simulink model "requirements"  (R2022a)
settings: Solver=FixedStepAuto  StartTime=0.0  StopTime=10.0  FixedStep=1e-3  RelTol=1e-3  EnableMultiTasking=on
settings Model: ExtModeTrigDuration=5  Creator=zaree  LastModifiedBy=zaree
settings OptimizationCC: EnhancedBackFolding=on  PassReuseOutputArgsAs=Individual arguments  ZeroExternalMemoryAtStartup=off  ZeroInternalMemoryAtStartup=off  MaxStackSize=64  OptimizeBlockOrder=speed  DifferentSizesBufferReuse=on  OptimizationCustomize=off  EfficientTunableParamExpr=on
settings DebuggingCC: ParameterTunabilityLossMsg=error
settings HardwareCC: ProdBitPerPointer=32  ProdBitPerSizeT=32  ProdBitPerPtrDiffT=32  ProdLargestAtomicInteger=Long  ProdLargestAtomicFloat=Double  ProdWordSize=32  ProdHWDeviceType=ARM Compatible->ARM Cortex
settings SFSimCC: MATLABDynamicMemAlloc=off
settings RTWCC: SystemTargetFile=ert.tlc  HardwareBoard=NXP FRDM-K64F  TLCOptions="-aInlineSetEventsForThisBaseRateFcn=TLC_FALSE -aSuppressMultiTaskScheduler=TLC_FALSE  -aRateBasedStepFcn=0"  TemplateMakefile=ert_default_tmf  Toolchain=GNU Tools for ARM Embedded Processors
settings CodeAppCC: ForceParamTrailComments=on  IgnoreCustomStorageClasses=off  OperatorAnnotations=on  SimulinkDataObjDesc=on  SFDataObjDesc=on  InsertBlockDesc=on
settings ERTTargetCC: ExtModeTransport=4  ExtModeMexFile=sendToCommService

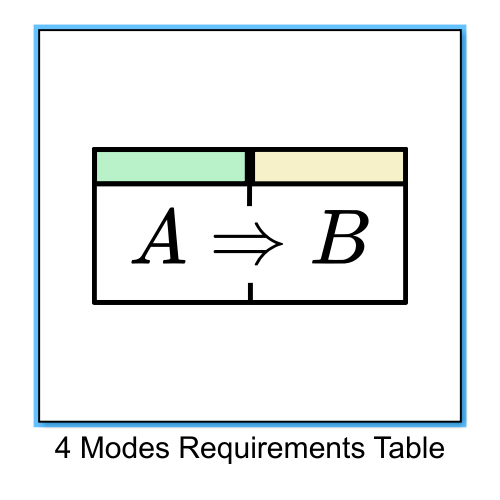
[thumbnail: Simulink's stored preview of the top-level diagram]
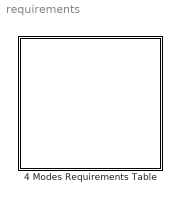
== system requirements ==
  4 Modes Requirements Table : Requirements Table  TreatAsAtomicUnit=on

== stateflow chart requirements/4 Modes Requirements Table ==
  (default) -> (junction 1073742873)
  (junction 1073742873) -> (junction 1073742874) : {
      | % SF_REQ_REV_07
      | }
  (junction 1073742874) -> (junction 1073742876) : {
      | % HEADER_ASSIGNMENTS
      |
      | }
  (junction 1073742876) -> (junction 1073742878) : {
      | % START_A_4
      | }
  (junction 1073742878) -> (junction 1073742880) : {
      | }
  (junction 1073742880) -> (junction 1073742882)
  (junction 1073742882) -> (junction 1073742884) : {
      | }
  (junction 1073742884) -> (junction 1073742886) : {
      | % END_A_4
      | }
  (junction 1073742886) -> (junction 1073742888) : {
      | % START_R_1
      | }
  (junction 1073742888) -> (junction 1073742890) : {
      | }
  (junction 1073742890) -> (junction 1073742892)
  (junction 1073742892) -> (junction 1073742894) [order 1] : [duration((PACE_CHARGE_CTRL == 0) && (ATR_CHARGE_CTRL == 1) && (ATR_GND_CTRL == 0) && (PACE_GND_CTRL == 1) && (Z_ATR_CTRL == 0)) >= LRI-Atrial_Pulse_Width]
  (junction 1073742892) -> (junction 1073742900) [order 2]
  (junction 1073742894) -> (junction 1073742896) : {
      | reqtable_postcondition((PACE_CHARGE_CTRL == 1) && (ATR_PACE_CTRL == 0) && (ATR_GND_CTRL == 1) && (PACE_GND_CTRL == 1) && (Z_ATR_CTRL == 0), 'R:1');
      |
      |
      | }
  (junction 1073742896) -> (junction 1073742898) : {
      | }
  (junction 1073742898) -> (junction 1073742900)
  (junction 1073742900) -> (junction 1073742902)
  (junction 1073742902) -> (junction 1073742904) : {
      | % END_R_1
      | }
  (junction 1073742904) -> (junction 1073742906) : {
      | % START_R_7
      | }
  (junction 1073742906) -> (junction 1073742908) : {
      | }
  (junction 1073742908) -> (junction 1073742910)
  (junction 1073742910) -> (junction 1073742912) [order 1] : [duration((PACE_CHARGE_CTRL == 1) && (ATR_PACE_CTRL==0) && (ATR_GND_CTRL==1) && (PACE_GND_CTRL == 1) && (Z_ATR_CTRL == 0)) >= Atrial_Pulse_Width]
  (junction 1073742910) -> (junction 1073742918) [order 2]
  (junction 1073742912) -> (junction 1073742914) : {
      | reqtable_postcondition((PACE_CHARGE_CTRL == 0) && (ATR_CHARGE_CTRL == 1) && (ATR_GND_CTRL == 0) && (PACE_GND_CTRL == 1) && (Z_ATR_CTRL == 0), 'R:2');
      |
      |
      | }
  (junction 1073742914) -> (junction 1073742916) : {
      | }
  (junction 1073742916) -> (junction 1073742918)
  (junction 1073742918) -> (junction 1073742920)
  (junction 1073742920) -> (junction 1073742922) : {
      | % END_R_7
      | }
  (junction 1073742922) -> (junction 1073742924) : {
      | % START_R_10
      | }
  (junction 1073742924) -> (junction 1073742926) : {
      | }
  (junction 1073742926) -> (junction 1073742928)
  (junction 1073742928) -> (junction 1073742930) [order 1] : [duration((PACE_CHARGE_CTRL == 0) && (VENT_PACE_CTRL == 1) && (VENT_GND_CTRL == 0) && (PACE_GND_CTRL == 1) && (Z_VENT_CTRL == 0)) >= LRI-Ventricular_Pulse_Width]
  (junction 1073742928) -> (junction 1073742936) [order 2]
  (junction 1073742930) -> (junction 1073742932) : {
      | reqtable_postcondition((PACE_CHARGE_CTRL == 1) && (VENT_CHARGE_CTRL == 0) && (VENT_GND_CTRL == 1) && (PACE_GND_CTRL == 1) && (Z_VENT_CTRL == 0), 'R:3');
      |
      |
      | }
  (junction 1073742932) -> (junction 1073742934) : {
      | }
  (junction 1073742934) -> (junction 1073742936)
  (junction 1073742936) -> (junction 1073742938)
  (junction 1073742938) -> (junction 1073742940) : {
      | % END_R_10
      | }
  (junction 1073742940) -> (junction 1073742942) : {
      | % START_R_13
      | }
  (junction 1073742942) -> (junction 1073742944) : {
      | }
  (junction 1073742944) -> (junction 1073742946)
  (junction 1073742946) -> (junction 1073742948) [order 1] : [duration((PACE_CHARGE_CTRL == 1) && (VENT_PACE_CTRL == 0) && (VENT_GND_CTRL == 1) && (PACE_GND_CTRL == 1) && (Z_VENT_CTRL == 0)) >= Ventricular_Pulse_Width]
  (junction 1073742946) -> (junction 1073742954) [order 2]
  (junction 1073742948) -> (junction 1073742950) : {
      | reqtable_postcondition((PACE_CHARGE_CTRL == 0) && (VENT_CHARGE_CTRL == 1) && (VENT_GND_CTRL == 0) && (PACE_GND_CTRL == 1) && (Z_VENT_CTRL == 0), 'R:4');
      |
      |
      | }
  (junction 1073742950) -> (junction 1073742952) : {
      | }
  (junction 1073742952) -> (junction 1073742954)
  (junction 1073742954) -> (junction 1073742956)
  (junction 1073742956) -> (junction 1073742958) : {
      | % END_R_13
      | }
  (junction 1073742958) -> (junction 1073742960) : {
      | % START_R_22
      | }
  (junction 1073742960) -> (junction 1073742962) : {
      | }
  (junction 1073742962) -> (junction 1073742964)
  (junction 1073742964) -> (junction 1073742966) [order 1] : [duration((PACE_CHARGE_CTRL == 1) && (ATR_PACE_CTRL == 1) && (ATR_GND_CTRL == 0) && (PACE_GND_CTRL == 0 ) && (Z_ATR_CTRL == 0) && (ATR_CMP_DETECT ==1)) >= 2*ARP]
  (junction 1073742964) -> (junction 1073742972) [order 2]
  (junction 1073742966) -> (junction 1073742968) : {
      | reqtable_postcondition((PACE_CHARGE_CTRL == 1) && (ATR_PACE_CTRL == 1) && (ATR_GND_CTRL == 0) && (PACE_GND_CTRL == 0) && (Z_ATR_CTRL == 0) && (ATR_CMP_DETECT ==1), 'R:5');
      | SENSE
      |
      | }
  (junction 1073742968) -> (junction 1073742970) : {
      | }
  (junction 1073742970) -> (junction 1073742972)
  (junction 1073742972) -> (junction 1073742974)
  (junction 1073742974) -> (junction 1073742976) : {
      | % END_R_22
      | }
  (junction 1073742976) -> (junction 1073742978) : {
      | % START_R_25
      | }
  (junction 1073742978) -> (junction 1073742980) : {
      | }
  (junction 1073742980) -> (junction 1073742982)
  (junction 1073742982) -> (junction 1073742984) [order 1] : [duration((PACE_CHARGE_CTRL == 1) && (ATR_PACE_CTRL == 1) && (ATR_GND_CTRL == 0) && (PACE_GND_CTRL == 0) && (Z_ATR_CTRL == 0) && (ATR_CMP_DETECT ==0)) >= LRI]
  (junction 1073742982) -> (junction 1073742990) [order 2]
  (junction 1073742984) -> (junction 1073742986) : {
      | reqtable_postcondition((PACE_CHARGE_CTRL == 0) && (ATR_PACE_CTRL == 1) && (ATR_GND_CTRL == 0) && (PACE_GND_CTRL == 1) && (Z_ATR_CTRL == 0) && (ATR_CMP_DETECT ==0), 'R:6');
      | PACE
      |
      | }
  (junction 1073742986) -> (junction 1073742988) : {
      | }
  (junction 1073742988) -> (junction 1073742990)
  (junction 1073742990) -> (junction 1073742992)
  (junction 1073742992) -> (junction 1073742994) : {
      | % END_R_25
      | }
  (junction 1073742994) -> (junction 1073742996) : {
      | % START_R_34
      | }
  (junction 1073742996) -> (junction 1073742998) : {
      | }
  (junction 1073742998) -> (junction 1073743000)
  (junction 1073743000) -> (junction 1073743002) [order 1] : [duration((PACE_CHARGE_CTRL == 0) && (ATR_PACE_CTRL == 1) && (ATR_GND_CTRL == 0) && (PACE_GND_CTRL == 1) && (Z_ATR_CTRL == 0) && (ATR_CMP_DETECT ==1)) >= Atrium_Pulse_Width]
  (junction 1073743000) -> (junction 1073743008) [order 2]
  (junction 1073743002) -> (junction 1073743004) : {
      | reqtable_postcondition((PACE_CHARGE_CTRL == 1) && (ATR_PACE_CTRL == 1) && (ATR_GND_CTRL == 0) && (PACE_GND_CTRL == 0 ) && (Z_ATR_CTRL == 0) && (ATR_CMP_DETECT ==1), 'R:7');
      | SENSE
      |
      | }
  (junction 1073743004) -> (junction 1073743006) : {
      | }
  (junction 1073743006) -> (junction 1073743008)
  (junction 1073743008) -> (junction 1073743010)
  (junction 1073743010) -> (junction 1073743012) : {
      | % END_R_34
      | }
  (junction 1073743012) -> (junction 1073743014) : {
      | % START_R_28
      | }
  (junction 1073743014) -> (junction 1073743016) : {
      | }
  (junction 1073743016) -> (junction 1073743018)
  (junction 1073743018) -> (junction 1073743020) [order 1] : [duration((PACE_CHARGE_CTRL == 1) && (VENT_PACE_CTRL == 1) && (VENT_GND_CTRL == 0) && (PACE_GND_CTRL == 0 ) && (Z_VENT_CTRL == 0) && (VENT_CMP_DETECT ==1)) >= 2*VRP]
  (junction 1073743018) -> (junction 1073743026) [order 2]
  (junction 1073743020) -> (junction 1073743022) : {
      | reqtable_postcondition((PACE_CHARGE_CTRL == 1) && (VENT_PACE_CTRL == 1) && (VENT_GND_CTRL == 0) && (PACE_GND_CTRL == 0) && (Z_VENT_CTRL == 0) && (VENT_CMP_DETECT ==1), 'R:8');
      | SENSE
      |
      | }
  (junction 1073743022) -> (junction 1073743024) : {
      | }
  (junction 1073743024) -> (junction 1073743026)
  (junction 1073743026) -> (junction 1073743028)
  (junction 1073743028) -> (junction 1073743030) : {
      | % END_R_28
      | }
  (junction 1073743030) -> (junction 1073743032) : {
      | % START_R_31
      | }
  (junction 1073743032) -> (junction 1073743034) : {
      | }
  (junction 1073743034) -> (junction 1073743036)
  (junction 1073743036) -> (junction 1073743038) [order 1] : [duration((PACE_CHARGE_CTRL == 1) && (VENT_PACE_CTRL == 1) && (VENT_GND_CTRL == 0) && (PACE_GND_CTRL == 0) && (Z_VENT_CTRL == 0) && (VENT_CMP_DETECT ==0)) >= LRI]
  (junction 1073743036) -> (junction 1073743044) [order 2]
  (junction 1073743038) -> (junction 1073743040) : {
      | reqtable_postcondition((PACE_CHARGE_CTRL == 0) && (VENT_PACE_CTRL == 1) && (VENT_GND_CTRL == 0) && (PACE_GND_CTRL == 1) && (Z_VENT_CTRL == 0) && (VENT_CMP_DETECT ==0), 'R:9');
      | PACE
      |
      | }
  (junction 1073743040) -> (junction 1073743042) : {
      | }
  (junction 1073743042) -> (junction 1073743044)
  (junction 1073743044) -> (junction 1073743046)
  (junction 1073743046) -> (junction 1073743048) : {
      | % END_R_31
      | }
  (junction 1073743048) -> (junction 1073743050) : {
      | % START_R_37
      | }
  (junction 1073743050) -> (junction 1073743052) : {
      | }
  (junction 1073743052) -> (junction 1073743054)
  (junction 1073743054) -> (junction 1073743056) [order 1] : [duration((PACE_CHARGE_CTRL == 0) && (VENT_PACE_CTRL == 1) && (VENT_GND_CTRL == 0) && (PACE_GND_CTRL == 1) && (Z_VENT_CTRL == 0) && (VENT_CMP_DETECT ==0)) >= Ventricular_Pulse_Width]
  (junction 1073743054) -> (junction 1073743062) [order 2]
  (junction 1073743056) -> (junction 1073743058) : {
      | reqtable_postcondition((PACE_CHARGE_CTRL == 1) && (VENT_PACE_CTRL == 1) && (VENT_GND_CTRL == 0) && (PACE_GND_CTRL == 0 ) && (Z_VENT_CTRL == 0) && (VENT_CMP_DETECT ==1), 'R:10');
      | SENSE
      |
      | }
  (junction 1073743058) -> (junction 1073743060) : {
      | }
  (junction 1073743060) -> (junction 1073743062)
  (junction 1073743062) -> (junction 1073743064)
  (junction 1073743064) -> (junction 1073743066) : {
      | % END_R_37
      | }
